simulink model "switch_subsystem"  (R2015b)
settings: Solver=FixedStepDiscrete  StartTime=0.0  StopTime=10.0  FixedStep=0.1  RelTol=1e-3
libraries: simulink x1
settings Model: Creator=studypc2  LastModifiedBy=admin-cs
settings DataIOCC: SaveFormat=Array  SignalLogging=off
settings OptimizationCC: ExpressionDepthLimit=2147483647
settings DebuggingCC: UnderspecifiedInitializationDetection=Classic  MergeDetectMultiDrivingBlocksExec=none  SolverPrmCheckMsg=warning  StateNameClashWarn=warning
settings HardwareCC: ProdBitPerPointer=32  ProdLargestAtomicFloat=None  ProdIntDivRoundTo=Undefined  ProdEndianess=Unspecified  ProdWordSize=32  ProdHWDeviceType=32-bit Generic
settings GRTTargetCC: GeneratePreprocessorConditionals=Disable all
settings ConfigComp: CovModelRefEnable=Off

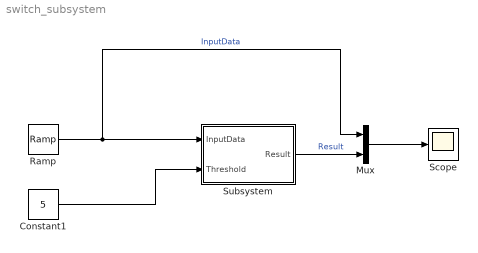
== system switch_subsystem ==
  Constant1 : Constant  Value=5
  Mux : Mux  Inputs=2
  Ramp : simulink/Sources/Ramp  slope=1  start=0  X0=0
  Scope : Scope
  Subsystem : Subsystem
  wires:
  Mux/1 -> Scope/1
  Ramp/1 -> Mux/1, Subsystem/1(InputData)  "InputData"
  Constant1/1 -> Subsystem/2(Threshold)
  Subsystem/1(Result) -> Mux/2  "Result"

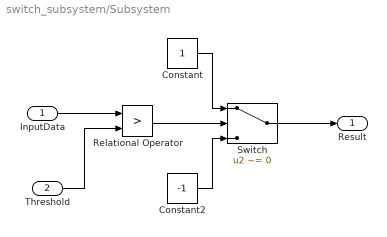
== system switch_subsystem/Subsystem ==
  InputData : Inport
  Threshold : Inport  Port=2
  Constant : Constant
  Constant2 : Constant  Value=-1
  Relational Operator : RelationalOperator  Operator=>  OutDataTypeStr=boolean
  Switch : Switch  Criteria=u2 ~= 0
  Result : Outport
  wires:
  Constant/1 -> Switch/1
  Relational Operator/1 -> Switch/2
  Constant2/1 -> Switch/3
  Threshold/1 -> Relational Operator/2
  Switch/1 -> Result/1
  InputData/1 -> Relational Operator/1
